simulink model "bh_zaz"  (R2019b)
settings: Solver=ode15s  StartTime=0.0  StopTime=6  FixedStep=0.001  MaxStep=0.1  RelTol=1e-5  AbsTol=1e-5  EnableMultiTasking=on
values from neighbouring files (symbols this model uses):
  L1 = 0.4    [bh_4bar_kin_z_analysis_CLS.m]
  L2 = 1.4    [bh_4bar_kin_z_analysis_CLS.m]
  L3 = 1.2    [bh_4bar_kin_z_analysis_CLS.m]
  N = length(THE_DEG_ANG_VEC)    [bh_4bar_kin_z_analysis_CLS.m]
  X = my_stuff_T.theta_deg_vec    [bh_4bar_kin_z_analysis_CLS.m]
undefined symbols (not defined in the file or in its folder): alpha_0_rad, alpha_dot_0_rad, g, H, I_G1, I_G2, I_G3, m1, m2, m3, phi_0_rad, phi_dot_0_rad, theta_0_rad, theta_dot_0_rad, W, Y, Z
libraries: nesl_utility x20, sm_lib x15, bh_4bar_SL_LIB x6, simulink_extras x5
(part 1 of 2)
settings Model: EnablePacing=on  Creator=bhorton  LastModifiedBy=bhorton
settings DataIOCC: LimitDataPoints=on  ReturnWorkspaceOutputs=off
settings OptimizationCC: LifeSpan=inf
settings DebuggingCC: AllowSymbolicDim=off  PregeneratedLibrarySubsystemCodeDiagnostic=none  SFUnexpectedBacktrackingDiag=warning  SFNoUnconditionalDefaultTransitionDiag=warning  SFExecutionAtInitializationDiag=none  ArithmeticOperatorsInVariantConditions=warning
settings SFSimCC: SimUseLocalCustomCode=off  CustomCodeUndefinedFunction=UseInterfaceOnly
settings RTWCC: RTWUseLocalCustomCode=off
settings CodeAppCC: StateflowObjectComments=on
settings GRTTargetCC: TargetLangStandard=C89/C90 (ANSI)  GeneratePreprocessorConditionals=Disable all
settings ConfigComp: CovMetricSettings=dw  CovHtmlReporting=on  CovSaveCumulativeToWorkspaceVar=on  CovSaveSingleToWorkspaceVar=on  CovExternalEMLEnable=off  CovSFcnEnable=off
settings SimscapeCC: SimscapeNominalValues="[{\"value\":\"10\",\"unit\":\"V\"},{\"value\":\"1\",\"unit\":\"A\"},{\"value\":\"10\",\"unit\":\"N*m\"},{\"value\":\"10\",\"unit\":\"bar\"},{\"value\":\"100\",\"unit\":\"kJ/kg\"},{\"value\":\"1\",\"unit\":\"kW\"},{\"value\":\"300\",\"unit\":\"K\"},{\"value\":\"100\",\"unit\":\"cm^3/s\"},{\"value\":\"1\",\"unit\":\"kN\"},{\"value\":\"1\",\"unit\":\"g/cm^3\"},{\"value\":\"1\",\"unit\":\"l\"},{\"value\":\"1\",\"unit\":\"cm^2\"},{\"value\":\"60\",\"unit\":\"Hz\"}]"  SimscapeLogType=all  SimscapeLogDataHistory=10000
settings ConfigurationSet: Description=SimMechanics 2G
settings ExplorerConfigSet: InternalSimMechanicsExplorerSettings="<ExplorerConfiguration><canonicalview>default</canonicalview><AnimationSetting><BasePlaybackSpeed>1.0</BasePlaybackSpeed><PlaybackSpeedFactor>1.0</PlaybackSpeedFactor></AnimationSetting><TilePanel><TileInfo><Tiles Columns=\"1\" Count=\"1\" Rows=\"1\"><Column Weight=\"1\"/><Row Weight=\"1\"/><Tile Height=\"1\" Width=\"1\" X=\"0\" Y=\"0\"/></Tiles></TileInfo><SceneInfo><SceneViewer><BGColor><R>0.60000002384185791</R><G>0.60000002384185791</G><B>0.60000002384185791</B></BGColor><Camera><DoPerspective>off</DoPerspective><Position><X>0.674057005362880823</X><Y>0.451513124756151407</Y><Z>1.11774542835223722</Z></Position><Center><X>0.674057005362880823</X><Y>0.451513124756151407</Y><Z>-0.00200006458294343936</Z></Center><Up><X>0</X><Y>1</Y><Z>-0</Z></Up><ViewLimDist>1</ViewLimDist><YLim>0.872355052534568132</YLim><XLim>1.30853257880185225</XLim></Camera></SceneViewer></SceneInfo></TilePanel><MechEditorPanel><Cameras/><GfxPanelCameraMap/><VideoCreator><PlaybackSpeedRatio>1.0</PlaybackSpeedRatio><FrameRate>30</FrameRate><VideoFormat>Motion JPEG AVI</VideoFormat><FrameSize>auto</FrameSize></VideoCreator></MechEditorPanel></ExplorerConfiguration>"

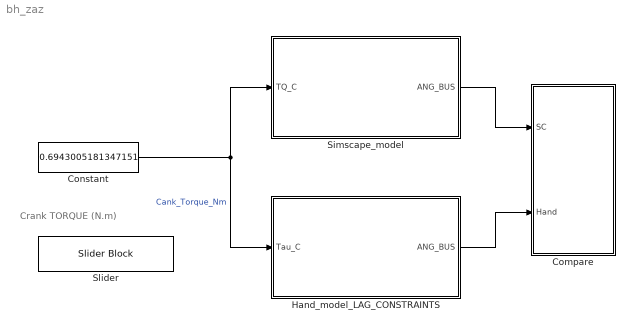
== system bh_zaz ==
  note: Crank TORQUE (N.m)
  Compare : Subsystem
  Constant : Constant  Value=0.6943005181347151
  Hand_model_LAG_CONSTRAINTS : Subsystem
  Simscape_model : Subsystem
  Slider : SliderBlock  ScaleMax=1
  wires:
  Constant/1 -> Simscape_model/1(TQ_C), Hand_model_LAG_CONSTRAINTS/1(Tau_C)  "Cank_Torque_Nm"
  Simscape_model/1(ANG_BUS) -> Compare/1(SC)
  Hand_model_LAG_CONSTRAINTS/1(ANG_BUS) -> Compare/2(Hand)

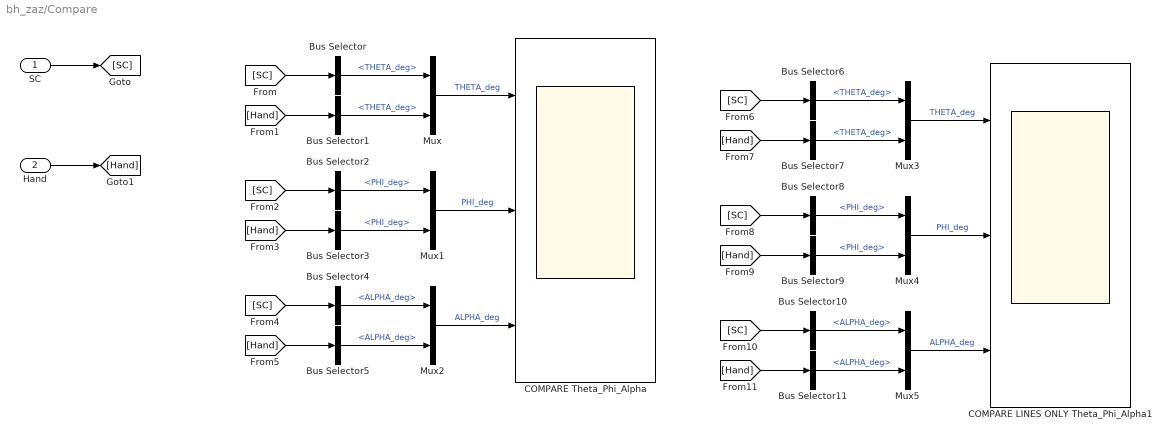
== system bh_zaz/Compare ==
  SC : Inport
  Hand : Inport  Port=2
  Bus Selector{,1,6..7} (4 alike) : BusSelector  OutputSignals=THETA_deg
  Bus Selector{4..5,10..11} (4 alike) : BusSelector  OutputSignals=ALPHA_deg
  Bus Selector{2..3,8..9} (4 alike) : BusSelector  OutputSignals=PHI_deg
  COMPARE LINES ONLY Theta_Phi_Alpha1 : Scope  NumInputPorts=3
  COMPARE Theta_Phi_Alpha : Scope  NumInputPorts=3
  Mux{,1..5} (6 alike) : Mux  Inputs=2
  wires:
  Hand/1 -> [Hand]
  SC/1 -> [SC]
  Mux/1 -> COMPARE Theta_Phi_Alpha/1  "THETA_deg"
  [SC] -> Bus Selector/1
  Bus Selector/1 -> Mux/1  "<THETA_deg>"
  [Hand] -> Bus Selector1/1
  Bus Selector1/1 -> Mux/2  "<THETA_deg>"
  Mux1/1 -> COMPARE Theta_Phi_Alpha/2  "PHI_deg"
  [SC] -> Bus Selector2/1
  Bus Selector3/1 -> Mux1/2  "<PHI_deg>"
  [Hand] -> Bus Selector3/1
  Bus Selector2/1 -> Mux1/1  "<PHI_deg>"
  Mux2/1 -> COMPARE Theta_Phi_Alpha/3  "ALPHA_deg"
  [Hand] -> Bus Selector5/1
  [SC] -> Bus Selector4/1
  Bus Selector5/1 -> Mux2/2  "<ALPHA_deg>"
  Bus Selector4/1 -> Mux2/1  "<ALPHA_deg>"
  Bus Selector10/1 -> Mux5/1  "<ALPHA_deg>"
  [Hand] -> Bus Selector11/1
  Mux5/1 -> COMPARE LINES ONLY Theta_Phi_Alpha1/3  "ALPHA_deg"
  Bus Selector11/1 -> Mux5/2  "<ALPHA_deg>"
  Mux4/1 -> COMPARE LINES ONLY Theta_Phi_Alpha1/2  "PHI_deg"
  [Hand] -> Bus Selector7/1
  Bus Selector8/1 -> Mux4/1  "<PHI_deg>"
  [SC] -> Bus Selector6/1
  Mux3/1 -> COMPARE LINES ONLY Theta_Phi_Alpha1/1  "THETA_deg"
  Bus Selector6/1 -> Mux3/1  "<THETA_deg>"
  [Hand] -> Bus Selector9/1
  [SC] -> Bus Selector8/1
  Bus Selector7/1 -> Mux3/2  "<THETA_deg>"
  [SC] -> Bus Selector10/1
  Bus Selector9/1 -> Mux4/2  "<PHI_deg>"

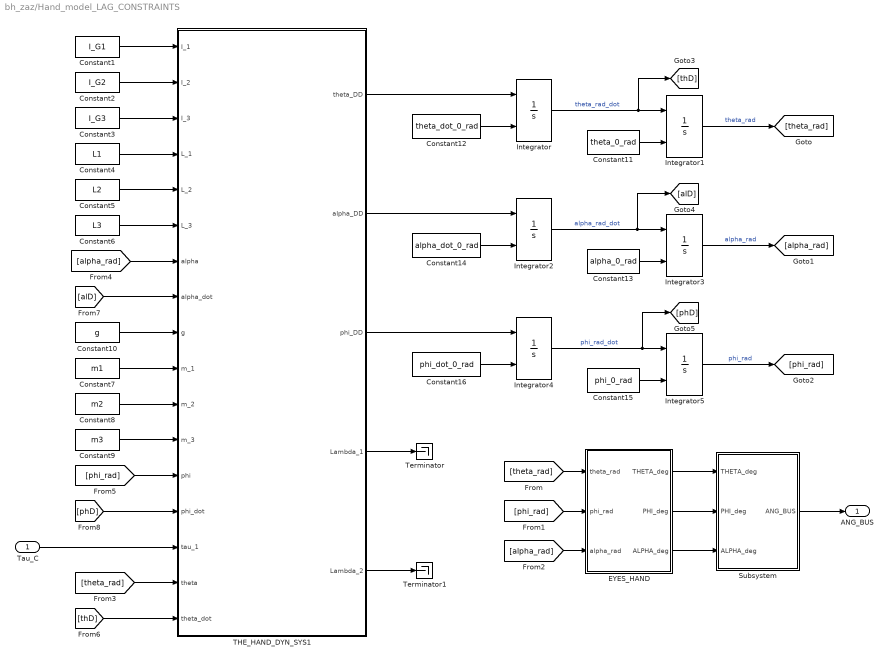
== system bh_zaz/Hand_model_LAG_CONSTRAINTS ==
  Tau_C : Inport
  Constant1 : Constant  Value=I_G1
  Constant10 : Constant  Value=g
  Constant11 : Constant  Value=theta_0_rad
  Constant12 : Constant  Value=theta_dot_0_rad
  Constant13 : Constant  Value=alpha_0_rad
  Constant14 : Constant  Value=alpha_dot_0_rad
  Constant15 : Constant  Value=phi_0_rad
  Constant16 : Constant  Value=phi_dot_0_rad
  Constant2 : Constant  Value=I_G2
  Constant3 : Constant  Value=I_G3
  Constant4 : Constant  Value=L1
  Constant5 : Constant  Value=L2
  Constant6 : Constant  Value=L3
  Constant7 : Constant  Value=m1
  Constant8 : Constant  Value=m2
  Constant9 : Constant  Value=m3
  EYES_HAND : Subsystem
  Integrator{,1..5} (6 alike) : Integrator  InitialConditionSource=external
  Subsystem : Subsystem
  THE_HAND_DYN_SYS1 : MATLAB Function  TreatAsAtomicUnit=on
  Terminator : Terminator
  Terminator1 : Terminator
  ANG_BUS : Outport  VectorParamsAs1DForOutWhenUnconnected=off
  wires:
  Constant7/1 -> THE_HAND_DYN_SYS1/10(m_1)
  Constant8/1 -> THE_HAND_DYN_SYS1/11(m_2)
  Integrator/1 -> [thD], Integrator1/1  "theta_rad_dot"
  Constant6/1 -> THE_HAND_DYN_SYS1/6(L_3)
  Integrator1/1 -> [theta_rad]  "theta_rad"
  Subsystem/1(ANG_BUS) -> ANG_BUS/1
  Constant5/1 -> THE_HAND_DYN_SYS1/5(L_2)
  EYES_HAND/2(PHI_deg) -> Subsystem/2(PHI_deg)
  EYES_HAND/1(THETA_deg) -> Subsystem/1(THETA_deg)
  EYES_HAND/3(ALPHA_deg) -> Subsystem/3(ALPHA_deg)
  [theta_rad] -> EYES_HAND/1(theta_rad)
  [phi_rad] -> EYES_HAND/2(phi_rad)
  THE_HAND_DYN_SYS1/1(theta_DD) -> Integrator/1
  [alpha_rad] -> EYES_HAND/3(alpha_rad)
  Constant3/1 -> THE_HAND_DYN_SYS1/3(I_3)
  Constant2/1 -> THE_HAND_DYN_SYS1/2(I_2)
  Constant4/1 -> THE_HAND_DYN_SYS1/4(L_1)
  Constant10/1 -> THE_HAND_DYN_SYS1/9(g)
  Constant9/1 -> THE_HAND_DYN_SYS1/12(m_3)
  Constant1/1 -> THE_HAND_DYN_SYS1/1(I_1)
  Tau_C/1 -> THE_HAND_DYN_SYS1/15(tau_1)
  Constant12/1 -> Integrator/2
  Constant11/1 -> Integrator1/2
  Integrator2/1 -> [alD], Integrator3/1  "alpha_rad_dot"
  THE_HAND_DYN_SYS1/2(alpha_DD) -> Integrator2/1
  Constant13/1 -> Integrator3/2
  Integrator3/1 -> [alpha_rad]  "alpha_rad"
  Constant14/1 -> Integrator2/2
  Constant15/1 -> Integrator5/2
  Integrator4/1 -> [phD], Integrator5/1  "phi_rad_dot"
  Integrator5/1 -> [phi_rad]  "phi_rad"
  Constant16/1 -> Integrator4/2
  THE_HAND_DYN_SYS1/3(phi_DD) -> Integrator4/1
  THE_HAND_DYN_SYS1/4(Lambda_1) -> Terminator/1
  THE_HAND_DYN_SYS1/5(Lambda_2) -> Terminator1/1
  [theta_rad] -> THE_HAND_DYN_SYS1/16(theta)
  [thD] -> THE_HAND_DYN_SYS1/17(theta_dot)
  [phD] -> THE_HAND_DYN_SYS1/14(phi_dot)
  [phi_rad] -> THE_HAND_DYN_SYS1/13(phi)
  [alD] -> THE_HAND_DYN_SYS1/8(alpha_dot)
  [alpha_rad] -> THE_HAND_DYN_SYS1/7(alpha)

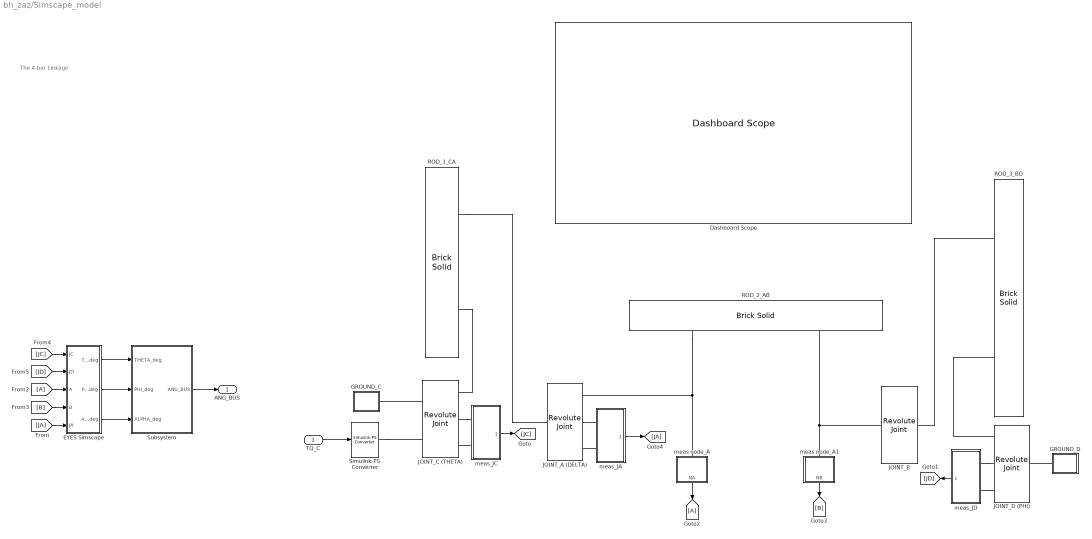
== system bh_zaz/Simscape_model ==
  note: The 4-bar Linkage
  TQ_C : Inport
  Dashboard Scope : DashboardScope
  EYES Simscape : Subsystem
  GROUND_C : Subsystem
  GROUND_D : Subsystem
  JOINT_A (DELTA) : sm_lib/Joints/Revolute Joint  JointMode=Normal  SenseConstraintForce=off  SenseConstraintForceX=off  SenseConstraintForceY=off  SenseConstraintForceZ=off  SenseConstraintTorque=off  SenseConstraintTorqueX=off  SenseConstraintTorqueY=off  SenseConstraintTorqueZ=off  SenseTotalForce=off  SenseTotalForceX=off  SenseTotalForceY=off  SenseTotalForceZ=off  SenseTotalTorque=off  SenseTotalTorqueX=off  SenseTotalTorqueY=off  SenseTotalTorqueZ=off  CompositeWrenchDir=FollowerOnBase  CompositeWrenchFrame=BaseFrame  EquilibriumPosition=0  EquilibriumPositionUnits=deg  SpringStiffness=0  SpringStiffnessUnits=N*m/deg  DampingCoefficient=0  DampingCoefficientUnits=N*m/(deg/s)  TorqueActuationMode=NoTorque  MotionActuationMode=ComputedMotion  SensePosition=on  SenseVelocity=on  SenseAcceleration=off  SenseTorqueForce=off  SenseLowerLimitTorqueForce=off  SenseUpperLimitTorqueForce=off  LowerLimitSpecify=off  LowerLimitBound=-90  LowerLimitBoundUnits=deg  LowerLimitStiffness=1e4  LowerLimitStiffnessUnits=N*m/deg  LowerLimitDamping=10  LowerLimitDampingUnits=N*m/(deg/s)  LowerLimitTransitionRegionWidth=0.1  LowerLimitTransitionRegionWidthUnits=deg  UpperLimitSpecify=off  UpperLimitBound=90  UpperLimitBoundUnits=deg  UpperLimitStiffness=1e4  UpperLimitStiffnessUnits=N*m/deg  UpperLimitDamping=10  UpperLimitDampingUnits=N*m/(deg/s)  UpperLimitTransitionRegionWidth=0.1  UpperLimitTransitionRegionWidthUnits=deg  PositionTargetSpecify=off  PositionTargetPriority=High  PositionTargetValue=0  PositionTargetValueUnits=deg  VelocityTargetSpecify=off  VelocityTargetPriority=High  VelocityTargetValue=0  VelocityTargetValueUnits=deg/s
  JOINT_B : sm_lib/Joints/Revolute Joint  JointMode=Normal  SenseConstraintForce=off  SenseConstraintForceX=off  SenseConstraintForceY=off  SenseConstraintForceZ=off  SenseConstraintTorque=off  SenseConstraintTorqueX=off  SenseConstraintTorqueY=off  SenseConstraintTorqueZ=off  SenseTotalForce=off  SenseTotalForceX=off  SenseTotalForceY=off  SenseTotalForceZ=off  SenseTotalTorque=off  SenseTotalTorqueX=off  SenseTotalTorqueY=off  SenseTotalTorqueZ=off  CompositeWrenchDir=FollowerOnBase  CompositeWrenchFrame=BaseFrame  EquilibriumPosition=0  EquilibriumPositionUnits=deg  SpringStiffness=0  SpringStiffnessUnits=N*m/deg  DampingCoefficient=0  DampingCoefficientUnits=N*m/(deg/s)  TorqueActuationMode=NoTorque  MotionActuationMode=ComputedMotion  SensePosition=off  SenseVelocity=off  SenseAcceleration=off  SenseTorqueForce=off  SenseLowerLimitTorqueForce=off  SenseUpperLimitTorqueForce=off  LowerLimitSpecify=off  LowerLimitBound=-90  LowerLimitBoundUnits=deg  LowerLimitStiffness=1e4  LowerLimitStiffnessUnits=N*m/deg  LowerLimitDamping=10  LowerLimitDampingUnits=N*m/(deg/s)  LowerLimitTransitionRegionWidth=0.1  LowerLimitTransitionRegionWidthUnits=deg  UpperLimitSpecify=off  UpperLimitBound=90  UpperLimitBoundUnits=deg  UpperLimitStiffness=1e4  UpperLimitStiffnessUnits=N*m/deg  UpperLimitDamping=10  UpperLimitDampingUnits=N*m/(deg/s)  UpperLimitTransitionRegionWidth=0.1  UpperLimitTransitionRegionWidthUnits=deg  PositionTargetSpecify=off  PositionTargetPriority=High  PositionTargetValue=0  PositionTargetValueUnits=deg  VelocityTargetSpecify=off  VelocityTargetPriority=High  VelocityTargetValue=0  VelocityTargetValueUnits=deg/s
  JOINT_C (THETA) : sm_lib/Joints/Revolute Joint  JointMode=Normal  SenseConstraintForce=off  SenseConstraintForceX=off  SenseConstraintForceY=off  SenseConstraintForceZ=off  SenseConstraintTorque=off  SenseConstraintTorqueX=off  SenseConstraintTorqueY=off  SenseConstraintTorqueZ=off  SenseTotalForce=off  SenseTotalForceX=off  SenseTotalForceY=off  SenseTotalForceZ=off  SenseTotalTorque=off  SenseTotalTorqueX=off  SenseTotalTorqueY=off  SenseTotalTorqueZ=off  CompositeWrenchDir=FollowerOnBase  CompositeWrenchFrame=BaseFrame  EquilibriumPosition=0  EquilibriumPositionUnits=deg  SpringStiffness=0  SpringStiffnessUnits=N*m/deg  DampingCoefficient=0  DampingCoefficientUnits=N*m/(deg/s)  TorqueActuationMode=InputTorque  MotionActuationMode=ComputedMotion  SensePosition=on  SenseVelocity=on  SenseAcceleration=off  SenseTorqueForce=off  SenseLowerLimitTorqueForce=off  SenseUpperLimitTorqueForce=off  LowerLimitSpecify=off  LowerLimitBound=-90  LowerLimitBoundUnits=deg  LowerLimitStiffness=1e4  LowerLimitStiffnessUnits=N*m/deg  LowerLimitDamping=10  LowerLimitDampingUnits=N*m/(deg/s)  LowerLimitTransitionRegionWidth=0.1  LowerLimitTransitionRegionWidthUnits=deg  UpperLimitSpecify=off  UpperLimitBound=90  UpperLimitBoundUnits=deg  UpperLimitStiffness=1e4  UpperLimitStiffnessUnits=N*m/deg  UpperLimitDamping=10  UpperLimitDampingUnits=N*m/(deg/s)  UpperLimitTransitionRegionWidth=0.1  UpperLimitTransitionRegionWidthUnits=deg  PositionTargetSpecify=on  PositionTargetPriority=High  PositionTargetValue=joints.C.ang_degs  PositionTargetValueUnits=deg  VelocityTargetSpecify=on  VelocityTargetPriority=High  VelocityTargetValue=joints.C.vel_degs  VelocityTargetValueUnits=deg/s
      settings: AttributesFormatString=|
      | init_pos =%<PositionTargetValue>
      | %<PositionTargetValueUnits>
      | init_VEL =
      | %<VelocityTargetValue>
      | %<VelocityTargetValueUnits>
  JOINT_D (PHI) : sm_lib/Joints/Revolute Joint  JointMode=Normal  SenseConstraintForce=off  SenseConstraintForceX=off  SenseConstraintForceY=off  SenseConstraintForceZ=off  SenseConstraintTorque=off  SenseConstraintTorqueX=off  SenseConstraintTorqueY=off  SenseConstraintTorqueZ=off  SenseTotalForce=off  SenseTotalForceX=off  SenseTotalForceY=off  SenseTotalForceZ=off  SenseTotalTorque=off  SenseTotalTorqueX=off  SenseTotalTorqueY=off  SenseTotalTorqueZ=off  CompositeWrenchDir=FollowerOnBase  CompositeWrenchFrame=BaseFrame  EquilibriumPosition=0  EquilibriumPositionUnits=deg  SpringStiffness=0  SpringStiffnessUnits=N*m/deg  DampingCoefficient=0  DampingCoefficientUnits=N*m/(deg/s)  TorqueActuationMode=NoTorque  MotionActuationMode=ComputedMotion  SensePosition=on  SenseVelocity=on  SenseAcceleration=off  SenseTorqueForce=off  SenseLowerLimitTorqueForce=off  SenseUpperLimitTorqueForce=off  LowerLimitSpecify=off  LowerLimitBound=-90  LowerLimitBoundUnits=deg  LowerLimitStiffness=1e4  LowerLimitStiffnessUnits=N*m/deg  LowerLimitDamping=10  LowerLimitDampingUnits=N*m/(deg/s)  LowerLimitTransitionRegionWidth=0.1  LowerLimitTransitionRegionWidthUnits=deg  UpperLimitSpecify=off  UpperLimitBound=90  UpperLimitBoundUnits=deg  UpperLimitStiffness=1e4  UpperLimitStiffnessUnits=N*m/deg  UpperLimitDamping=10  UpperLimitDampingUnits=N*m/(deg/s)  UpperLimitTransitionRegionWidth=0.1  UpperLimitTransitionRegionWidthUnits=deg  PositionTargetSpecify=on  PositionTargetPriority=High  PositionTargetValue=joints.D.ang_degs  PositionTargetValueUnits=deg  VelocityTargetSpecify=off  VelocityTargetPriority=High  VelocityTargetValue=0  VelocityTargetValueUnits=deg/s
      settings: AttributesFormatString=|
      | init_pos =%<PositionTargetValue>
      | %<PositionTargetValueUnits>
  ROD_1_CA : sm_lib/Body Elements/Brick Solid  GraphicAmbientColor=[0.15 0.15 0.15 1.0]  BasedOnType=Density  BrickDimensions=[L1,H,W]  BrickDimensionUnits=m  CenterOfMass=[0 0 0]  CenterOfMassUnits=m  GraphicDiffuseColor=[1.0 0.4 0.6]  Density=density  DensityUnits=kg/m^3  DoExposeReferenceFrame=on  GraphicEmissiveColor=[0.0 0.0 0.0 1.0]  ExportEntireGeometry=off  SerializedFrames=<Frames><Frame><Id>Frame2</Id><Value><Name>A</Name><Origin><Source>GeometricFeature</Source><FeatureName>+z +x curve</FeatureName></Origin><PrimaryAxis><DefinedDirection>+Z</DefinedDirection><Source>ReferenceFrame</Source><SourceDirection>+Z</SourceDirection><FeatureName></FeatureName></PrimaryAxis><SecondaryAxis><DefinedDirection>+X</DefinedDirection><Source>ReferenceFrame</Source><SourceDirection>+X</SourceDirection><FeatureName></FeatureName></SecondaryAxis></Value></Frame><Frame><Id>Frame3</Id><Value><Name>C</Name><Origin><Source>GeometricFeature</Source><FeatureName>+z -x curve</FeatureName></Origin><PrimaryAxis><DefinedDirection>+Z</DefinedDirection><Source>ReferenceFrame</Source><SourceDirection>+Z</SourceDirection><FeatureName></FeatureName></PrimaryAxis><SecondaryAxis><DefinedDirection>+X</DefinedDirection><Source>ReferenceFrame</Source><SourceDirection>+X</SourceDirection><FeatureName></FeatureName></SecondaryAxis></Value></Frame></Frames>  MarkerShape=Sphere  MarkerSize=10  GraphicType=FromGeometry  InertiaType=CalculateFromGeometry  Mass=1  MassUnits=kg  MomentsOfInertia=[1 1 1]  MomentsOfInertiaUnits=kg*m^2  GraphicOpacity=1.0  ProductsOfInertia=[0 0 0]  ProductsOfInertiaUnits=kg*m^2  GraphicShininess=75  GraphicSpecularColor=[0.5 0.5 0.5 1.0]  GraphicVisPropType=SimpleVisualProperties
  ROD_2_AB : sm_lib/Body Elements/Brick Solid  GraphicAmbientColor=[0.15 0.15 0.15 1.0]  BasedOnType=Density  BrickDimensions=[L2,H,W]  BrickDimensionUnits=m  CenterOfMass=[0 0 0]  CenterOfMassUnits=m  GraphicDiffuseColor=[0.0 1.0 0.2]  Density=density  DensityUnits=kg/m^3  DoExposeReferenceFrame=on  GraphicEmissiveColor=[0.0 0.0 0.0 1.0]  ExportEntireGeometry=off  SerializedFrames=<Frames><Frame><Id>Frame1</Id><Value><Name>A</Name><Origin><Source>GeometricFeature</Source><FeatureName>+z -x curve</FeatureName></Origin><PrimaryAxis><DefinedDirection>+Z</DefinedDirection><Source>ReferenceFrame</Source><SourceDirection>+Z</SourceDirection><FeatureName></FeatureName></PrimaryAxis><SecondaryAxis><DefinedDirection>+X</DefinedDirection><Source>ReferenceFrame</Source><SourceDirection>+X</SourceDirection><FeatureName></FeatureName></SecondaryAxis></Value></Frame><Frame><Id>Frame2</Id><Value><Name>B</Name><Origin><Source>GeometricFeature</Source><FeatureName>+z +x curve</FeatureName></Origin><PrimaryAxis><DefinedDirection>+Z</DefinedDirection><Source>ReferenceFrame</Source><SourceDirection>+Z</SourceDirection><FeatureName></FeatureName></PrimaryAxis><SecondaryAxis><DefinedDirection>+X</DefinedDirection><Source>ReferenceFrame</Source><SourceDirection>+X</SourceDirection><FeatureName></FeatureName></SecondaryAxis></Value></Frame></Frames>  MarkerShape=Sphere  MarkerSize=10  GraphicType=FromGeometry  InertiaType=CalculateFromGeometry  Mass=1  MassUnits=kg  MomentsOfInertia=[1 1 1]  MomentsOfInertiaUnits=kg*m^2  GraphicOpacity=1.0  ProductsOfInertia=[0 0 0]  ProductsOfInertiaUnits=kg*m^2  GraphicShininess=75  GraphicSpecularColor=[0.5 0.5 0.5 1.0]  GraphicVisPropType=SimpleVisualProperties
  ROD_3_BD : sm_lib/Body Elements/Brick Solid  GraphicAmbientColor=[0.15 0.15 0.15 1.0]  BasedOnType=Density  BrickDimensions=[L3,H,W]  BrickDimensionUnits=m  CenterOfMass=[0 0 0]  CenterOfMassUnits=m  GraphicDiffuseColor=[0.2 0.2 1.0]  Density=density  DensityUnits=kg/m^3  DoExposeReferenceFrame=on  GraphicEmissiveColor=[0.0 0.0 0.0 1.0]  ExportEntireGeometry=off  SerializedFrames=<Frames><Frame><Id>Frame1</Id><Value><Name>B</Name><Origin><Source>GeometricFeature</Source><FeatureName>+z +x curve</FeatureName></Origin><PrimaryAxis><DefinedDirection>+Z</DefinedDirection><Source>ReferenceFrame</Source><SourceDirection>+Z</SourceDirection><FeatureName></FeatureName></PrimaryAxis><SecondaryAxis><DefinedDirection>+X</DefinedDirection><Source>ReferenceFrame</Source><SourceDirection>+X</SourceDirection><FeatureName></FeatureName></SecondaryAxis></Value></Frame><Frame><Id>Frame2</Id><Value><Name>D</Name><Origin><Source>GeometricFeature</Source><FeatureName>+z -x curve</FeatureName></Origin><PrimaryAxis><DefinedDirection>+Z</DefinedDirection><Source>ReferenceFrame</Source><SourceDirection>+Z</SourceDirection><FeatureName></FeatureName></PrimaryAxis><SecondaryAxis><DefinedDirection>+X</DefinedDirection><Source>ReferenceFrame</Source><SourceDirection>+X</SourceDirection><FeatureName></FeatureName></SecondaryAxis></Value></Frame></Frames>  MarkerShape=Sphere  MarkerSize=10  GraphicType=FromGeometry  InertiaType=CalculateFromGeometry  Mass=1  MassUnits=kg  MomentsOfInertia=[1 1 1]  MomentsOfInertiaUnits=kg*m^2  GraphicOpacity=1.0  ProductsOfInertia=[0 0 0]  ProductsOfInertiaUnits=kg*m^2  GraphicShininess=75  GraphicSpecularColor=[0.5 0.5 0.5 1.0]  GraphicVisPropType=SimpleVisualProperties
  Simulink-PS Converter : nesl_utility/Simulink-PS Converter  PhysicalDomain=network_engine_domain  SubClassName=ps_input  LeftPortType=input  RightPortType=output  PseudoPeriodic=off  Frequencies=[]  NoiseDistribution=none  NoiseParameters=[]  Unit=N*m  AffineConversion=off  FilteringAndDerivatives=filter  SimscapeFilterOrder=1  InputFilterTimeConstant=0.001  UdotUserProvided=2
  Subsystem : Subsystem
  meas node_A : Subsystem
  meas node_A1 : Subsystem
  meas_JA : Subsystem
  meas_JC : Subsystem
  meas_JD : Subsystem
  ANG_BUS : Outport  VectorParamsAs1DForOutWhenUnconnected=off
  wires:
  [JC] -> EYES Simscape/1(JC)
  meas_JC/1(PV_BUS) -> [JC]
  [JA] -> EYES Simscape/5(JA)
  [B] -> EYES Simscape/4(B)
  EYES Simscape/3(ALPHA_deg) -> Subsystem/3(ALPHA_deg)
  TQ_C/1 -> Simulink-PS Converter/1
  [JD] -> EYES Simscape/2(JD)
  [A] -> EYES Simscape/3(A)
  meas_JA/1(PV_BUS) -> [JA]
  EYES Simscape/1(THETA_deg) -> Subsystem/1(THETA_deg)
  meas_JD/1(PV_BUS) -> [JD]
  EYES Simscape/2(PHI_deg) -> Subsystem/2(PHI_deg)
  Subsystem/1(ANG_BUS) -> ANG_BUS/1
  meas node_A/1(NA) -> [A]
  meas node_A1/1(NB) -> [B]
  connections:
  meas_JD/LConn2 -- JOINT_D (PHI)/RConn3
  JOINT_D (PHI)/RConn1 -- ROD_3_BD/LConn2
  JOINT_C (THETA)/LConn1 -- GROUND_C/RConn1
  meas_JA/LConn1 -- JOINT_A (DELTA)/RConn2
  meas_JD/LConn1 -- JOINT_D (PHI)/RConn2
  ROD_3_BD/LConn1 -- JOINT_B/RConn1
  meas_JA/LConn2 -- JOINT_A (DELTA)/RConn3
  GROUND_D/RConn1 -- JOINT_D (PHI)/LConn1
  JOINT_C (THETA)/RConn2 -- meas_JC/LConn1
  ROD_2_AB/LConn1 -- meas node_A/LConn1 -- JOINT_A (DELTA)/RConn1
  ROD_1_CA/LConn2 -- JOINT_C (THETA)/RConn1
  Simulink-PS Converter/RConn1 -- JOINT_C (THETA)/LConn2
  meas_JC/LConn2 -- JOINT_C (THETA)/RConn3
  ROD_1_CA/LConn1 -- JOINT_A (DELTA)/LConn1
  JOINT_B/LConn1 -- meas node_A1/LConn1 -- ROD_2_AB/LConn2

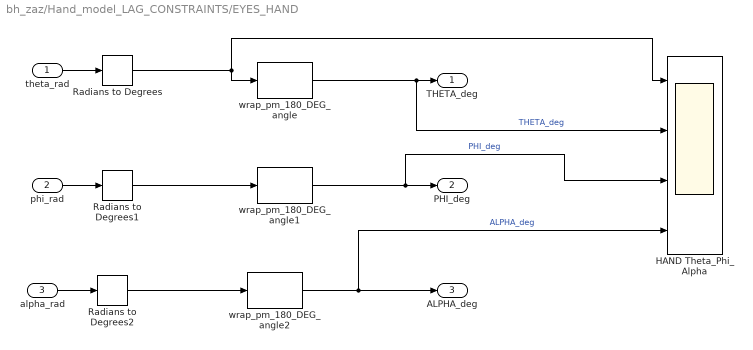
== system bh_zaz/Hand_model_LAG_CONSTRAINTS/EYES_HAND ==
  theta_rad : Inport
  phi_rad : Inport  Port=2
  alpha_rad : Inport  Port=3
  HAND Theta_Phi_Alpha : Scope  NumInputPorts=4
  Radians to Degrees : simulink_extras/Transformations/Radians to Degrees
  Radians to Degrees1 : simulink_extras/Transformations/Radians to Degrees
  Radians to Degrees2 : simulink_extras/Transformations/Radians to Degrees
  wrap_pm_180_DEG_angle : bh_4bar_SL_LIB/4bar_basics/wrap_pm_180_DEG_angle  SystemSampleTime=-1  Latency=0  AutoFrameSizeCalculation=off
  wrap_pm_180_DEG_angle1 : bh_4bar_SL_LIB/4bar_basics/wrap_pm_180_DEG_angle  SystemSampleTime=-1  Latency=0  AutoFrameSizeCalculation=off
  wrap_pm_180_DEG_angle2 : bh_4bar_SL_LIB/4bar_basics/wrap_pm_180_DEG_angle  SystemSampleTime=-1  Latency=0  AutoFrameSizeCalculation=off
  THETA_deg : Outport  VectorParamsAs1DForOutWhenUnconnected=off
  PHI_deg : Outport  Port=2  VectorParamsAs1DForOutWhenUnconnected=off
  ALPHA_deg : Outport  Port=3  VectorParamsAs1DForOutWhenUnconnected=off
  wires:
  theta_rad/1 -> Radians to Degrees/1
  alpha_rad/1 -> Radians to Degrees2/1
  phi_rad/1 -> Radians to Degrees1/1
  Radians to Degrees/1 -> wrap_pm_180_DEG_angle/1, HAND Theta_Phi_Alpha/1
  Radians to Degrees1/1 -> wrap_pm_180_DEG_angle1/1
  Radians to Degrees2/1 -> wrap_pm_180_DEG_angle2/1
  wrap_pm_180_DEG_angle/1 -> HAND Theta_Phi_Alpha/2, THETA_deg/1  "THETA_deg"
  wrap_pm_180_DEG_angle1/1 -> HAND Theta_Phi_Alpha/3, PHI_deg/1  "PHI_deg"
  wrap_pm_180_DEG_angle2/1 -> HAND Theta_Phi_Alpha/4, ALPHA_deg/1  "ALPHA_deg"

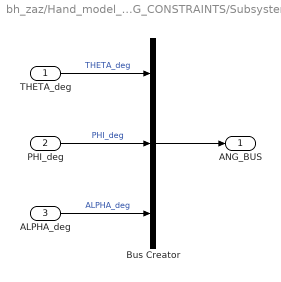
== system bh_zaz/Hand_model_LAG_CONSTRAINTS/Subsystem ==
  THETA_deg : Inport
  PHI_deg : Inport  Port=2
  ALPHA_deg : Inport  Port=3
  Bus Creator : BusCreator  Inputs=3
  ANG_BUS : Outport  VectorParamsAs1DForOutWhenUnconnected=off
  wires:
  ALPHA_deg/1 -> Bus Creator/3  "ALPHA_deg"
  PHI_deg/1 -> Bus Creator/2  "PHI_deg"
  THETA_deg/1 -> Bus Creator/1  "THETA_deg"
  Bus Creator/1 -> ANG_BUS/1

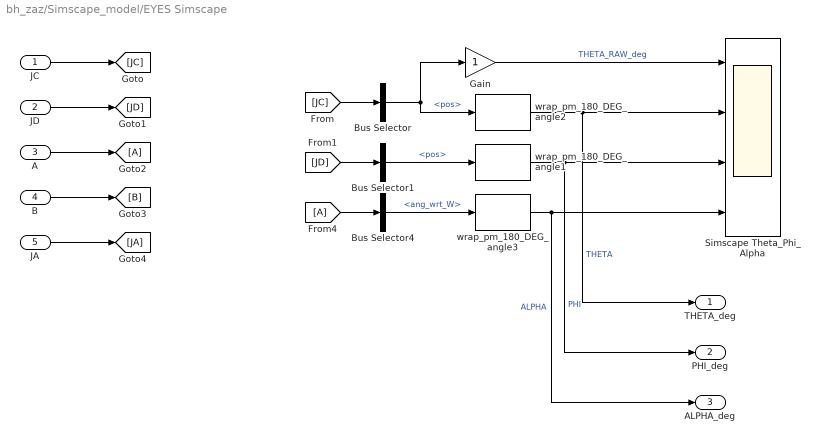
== system bh_zaz/Simscape_model/EYES Simscape ==
  JC : Inport
  JD : Inport  Port=2
  A : Inport  Port=3
  B : Inport  Port=4
  JA : Inport  Port=5
  Bus Selector : BusSelector  OutputSignals=pos
  Bus Selector1 : BusSelector  OutputSignals=pos
  Bus Selector4 : BusSelector  OutputSignals=ang_wrt_W
  Gain : Gain
  Simscape Theta_Phi_Alpha : Scope  NumInputPorts=4
  wrap_pm_180_DEG_angle1 : bh_4bar_SL_LIB/4bar_basics/wrap_pm_180_DEG_angle  SystemSampleTime=-1  Latency=0  AutoFrameSizeCalculation=off
  wrap_pm_180_DEG_angle2 : bh_4bar_SL_LIB/4bar_basics/wrap_pm_180_DEG_angle  SystemSampleTime=-1  Latency=0  AutoFrameSizeCalculation=off
  wrap_pm_180_DEG_angle3 : bh_4bar_SL_LIB/4bar_basics/wrap_pm_180_DEG_angle  SystemSampleTime=-1  Latency=0  AutoFrameSizeCalculation=off
  THETA_deg : Outport  VectorParamsAs1DForOutWhenUnconnected=off
  PHI_deg : Outport  Port=2  VectorParamsAs1DForOutWhenUnconnected=off
  ALPHA_deg : Outport  Port=3  VectorParamsAs1DForOutWhenUnconnected=off
  wires:
  B/1 -> [B]
  A/1 -> [A]
  JD/1 -> [JD]
  JC/1 -> [JC]
  [JD] -> Bus Selector1/1
  [JC] -> Bus Selector/1
  Bus Selector/1 -> wrap_pm_180_DEG_angle2/1, Gain/1  "<pos>"
  [A] -> Bus Selector4/1
  wrap_pm_180_DEG_angle2/1 -> THETA_deg/1, Simscape Theta_Phi_Alpha/2  "THETA"
  wrap_pm_180_DEG_angle1/1 -> PHI_deg/1, Simscape Theta_Phi_Alpha/3  "PHI"
  JA/1 -> [JA]
  wrap_pm_180_DEG_angle3/1 -> ALPHA_deg/1, Simscape Theta_Phi_Alpha/4  "ALPHA"
  Gain/1 -> Simscape Theta_Phi_Alpha/1  "THETA_RAW_deg"
  Bus Selector1/1 -> wrap_pm_180_DEG_angle1/1  "<pos>"
  Bus Selector4/1 -> wrap_pm_180_DEG_angle3/1  "<ang_wrt_W>"

== system bh_zaz/Simscape_model/GROUND_C ==
  Mechanism Configuration : sm_lib/Utilities/Mechanism Configuration  UniformGravity=Constant  GravityVector="[0 -g  0]"  GravityUnits=m/s^2  LinearizationDelta=0.001
  Solver Configuration : nesl_utility/Solver Configuration  PhysicalDomain=network_engine_domain  SubClassName=solver  LeftPortType=input  RightPortType=generic  Tones=[]  Harmonics=[]  SimulateNoise=off  Profile=off  UseLocalSampling=off  EnableSwitchedLinearOptims=on  FrequencyDomain=off  UseCCode=off  RelTol=0.001  AbsTol=1e-06  MinStep=1e-09  ToWorkspace=off  RevertToSquareIcSolve=off  NumHomotopyIterations=100  PhasorMode=off  PhasorModeNumHarmonics=1  DoDC=off  ResidualTolerance=1e-09  UseLocalSolver=off  LocalSolverChoice=NE_BACKWARD_EULER_ADVANCER  LocalSolverSampleTime=0.001  DoFixedCost=off  MaxNonlinIter=3  MaxModeIter=2  LinearAlgebra=Sparse  EquationFormulation=NE_TIME_EF  DelaysMemoryBudget=1024  AutomaticFiltering=on  FilteringTimeConstant=0.001  PartitionStorageMethod=AS_NEEDED  PartitionMemoryBudget=1024  PartitionMethod=FAST
  World Frame : sm_lib/Frames and Transforms/World Frame
  Conn1 : PMIOPort  Side=Right
  connections:
  Solver Configuration/RConn1 -- Conn1/RConn1 -- Mechanism Configuration/RConn1 -- World Frame/RConn1

== system bh_zaz/Simscape_model/GROUND_D ==
  Rigid Transform : sm_lib/Frames and Transforms/Rigid Transform  TranslationMethod=StandardAxis  TranslationStandardOffset=L4  TranslationLengthUnit=m  TranslationStandardAxis=+X  TranslationCartesianOffset=[0 0 0]  TranslationROffset=0  TranslationROffsetUnits=m  TranslationZOffset=0  TranslationZOffsetUnits=m  TranslationThetaOffset=0  TranslationThetaOffsetUnits=deg  RotationMethod=None  RotationAngleUnits=deg  RotationStandardAxis=+Z  RotationAngle=0.0  RotationArbitraryAxis=[0 0 1]  FollAlignAxisA=+X  BaseAlignAxisA=+Y  FollAlignAxisB=+Y  BaseAlignAxisB=+Z  RotationSequenceAxes=FollowerAxes  RotationSequence=XYX  RotationSequenceAngles=[0 0 0]  RotationSequenceAnglesUnits=deg  RotationMatrix=[1 0 0; 0 1 0; 0 0 1]
  World Frame1 : sm_lib/Frames and Transforms/World Frame
  Conn1 : PMIOPort  Side=Right
  connections:
  Rigid Transform/LConn1 -- World Frame1/RConn1
  Rigid Transform/RConn1 -- Conn1/RConn1

== system bh_zaz/Simscape_model/Subsystem ==
  THETA_deg : Inport
  PHI_deg : Inport  Port=2
  ALPHA_deg : Inport  Port=3
  Bus Creator : BusCreator  Inputs=3
  ANG_BUS : Outport  VectorParamsAs1DForOutWhenUnconnected=off
  wires:
  ALPHA_deg/1 -> Bus Creator/3  "ALPHA_deg"
  PHI_deg/1 -> Bus Creator/2  "PHI_deg"
  THETA_deg/1 -> Bus Creator/1  "THETA_deg"
  Bus Creator/1 -> ANG_BUS/1

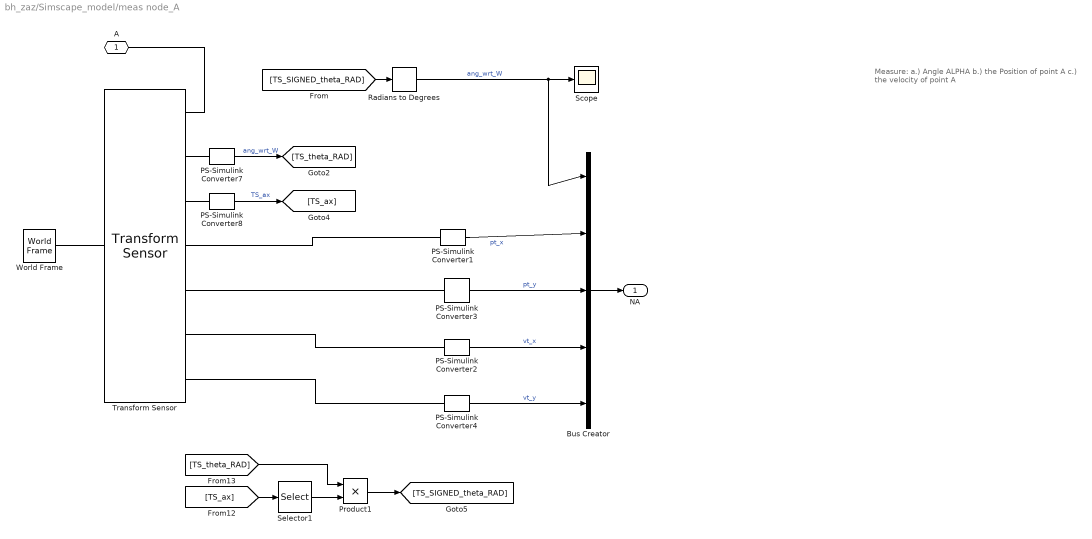
== system bh_zaz/Simscape_model/meas node_A ==
  note: Measure:
      | a.) Angle ALPHA
      | b.) the Position of point A
      | c.) the velocity of point A
  Bus Creator : BusCreator  Inputs=5
  PS-Simulink Converter1 : nesl_utility/PS-Simulink Converter  PhysicalDomain=network_engine_domain  SubClassName=ps_output  LeftPortType=input  RightPortType=output  PseudoPeriodic=off  Frequencies=[]  Unit=m  AffineConversion=off
      settings: AttributesFormatString=UNITS=%<Unit>
  PS-Simulink Converter2 : nesl_utility/PS-Simulink Converter  PhysicalDomain=network_engine_domain  SubClassName=ps_output  LeftPortType=input  RightPortType=output  PseudoPeriodic=off  Frequencies=[]  Unit=m/s  AffineConversion=off
      settings: AttributesFormatString=UNITS=%<Unit>
  PS-Simulink Converter3 : nesl_utility/PS-Simulink Converter  PhysicalDomain=network_engine_domain  SubClassName=ps_output  LeftPortType=input  RightPortType=output  PseudoPeriodic=off  Frequencies=[]  Unit=m  AffineConversion=off
      settings: AttributesFormatString=UNITS=%<Unit>
  PS-Simulink Converter4 : nesl_utility/PS-Simulink Converter  PhysicalDomain=network_engine_domain  SubClassName=ps_output  LeftPortType=input  RightPortType=output  PseudoPeriodic=off  Frequencies=[]  Unit=m/s  AffineConversion=off
      settings: AttributesFormatString=UNITS=%<Unit>
  PS-Simulink Converter7 : nesl_utility/PS-Simulink Converter  PhysicalDomain=network_engine_domain  SubClassName=ps_output  LeftPortType=input  RightPortType=output  PseudoPeriodic=off  Frequencies=[]  Unit=rad  AffineConversion=off
      settings: AttributesFormatString=UNITS=%<Unit>
  PS-Simulink Converter8 : nesl_utility/PS-Simulink Converter  PhysicalDomain=network_engine_domain  SubClassName=ps_output  LeftPortType=input  RightPortType=output  PseudoPeriodic=off  Frequencies=[]  Unit=1  AffineConversion=off
      settings: AttributesFormatString=UNITS=%<Unit>
  Product1 : Product
  Radians to Degrees : simulink_extras/Transformations/Radians to Degrees
  Scope : Scope
  Selector1 : Selector  InputPortWidth=3  IndexOptions=Index vector (dialog)  Indices=3  OutputSizes=1
  Transform Sensor : sm_lib/Frames and Transforms/Transform Sensor  MeasurementFrame=World  SenseAngle=on  SenseAxis=on  SenseAngle1=off  SenseAngle2=off  SenseAngle3=off  SenseQ=off  SenseR=off  SenseOmegaX=off  SenseOmegaY=off  SenseOmegaZ=off  SenseOmega1=off  SenseOmega2=off  SenseOmega3=off  SenseQDot=off  SenseRDot=off  SenseAlphaX=off  SenseAlphaY=off  SenseAlphaZ=off  SenseAlpha1=off  SenseAlpha2=off  SenseAlpha3=off  SenseQDDot=off  SenseRDDot=off  SenseX=on  SenseY=on  SenseZ=off  SenseRad=off  SenseAzim=off  SenseDist=off  SenseInc=off  SenseXDot=on  SenseYDot=on  SenseZDot=off  SenseRadDot=off  SenseAzimDot=off  SenseDistDot=off  SenseIncDot=off  SenseXDDot=off  SenseYDDot=off  SenseZDDot=off  SenseRadDDot=off  SenseAzimDDot=off  SenseDistDDot=off  SenseIncDDot=off
  World Frame : sm_lib/Frames and Transforms/World Frame
  A : PMIOPort  Side=Left
  NA : Outport  VectorParamsAs1DForOutWhenUnconnected=off
  wires:
  PS-Simulink Converter2/1 -> Bus Creator/4  "vt_x"
  Bus Creator/1 -> NA/1
  PS-Simulink Converter1/1 -> Bus Creator/2  "pt_x"
  PS-Simulink Converter4/1 -> Bus Creator/5  "vt_y"
  PS-Simulink Converter3/1 -> Bus Creator/3  "pt_y"
  Radians to Degrees/1 -> Bus Creator/1, Scope/1  "ang_wrt_W"
  [TS_theta_RAD] -> Product1/1
  [TS_ax] -> Selector1/1
  Product1/1 -> [TS_SIGNED_theta_RAD]
  Selector1/1 -> Product1/2
  PS-Simulink Converter7/1 -> [TS_theta_RAD]  "ang_wrt_W"
  PS-Simulink Converter8/1 -> [TS_ax]  "TS_ax"
  [TS_SIGNED_theta_RAD] -> Radians to Degrees/1
  connections:
  A/RConn1 -- Transform Sensor/RConn1
  Transform Sensor/LConn1 -- World Frame/RConn1
  Transform Sensor/RConn7 -- PS-Simulink Converter4/LConn1
  PS-Simulink Converter2/LConn1 -- Transform Sensor/RConn6
  PS-Simulink Converter3/LConn1 -- Transform Sensor/RConn5
  PS-Simulink Converter1/LConn1 -- Transform Sensor/RConn4
  PS-Simulink Converter7/LConn1 -- Transform Sensor/RConn2
  PS-Simulink Converter8/LConn1 -- Transform Sensor/RConn3

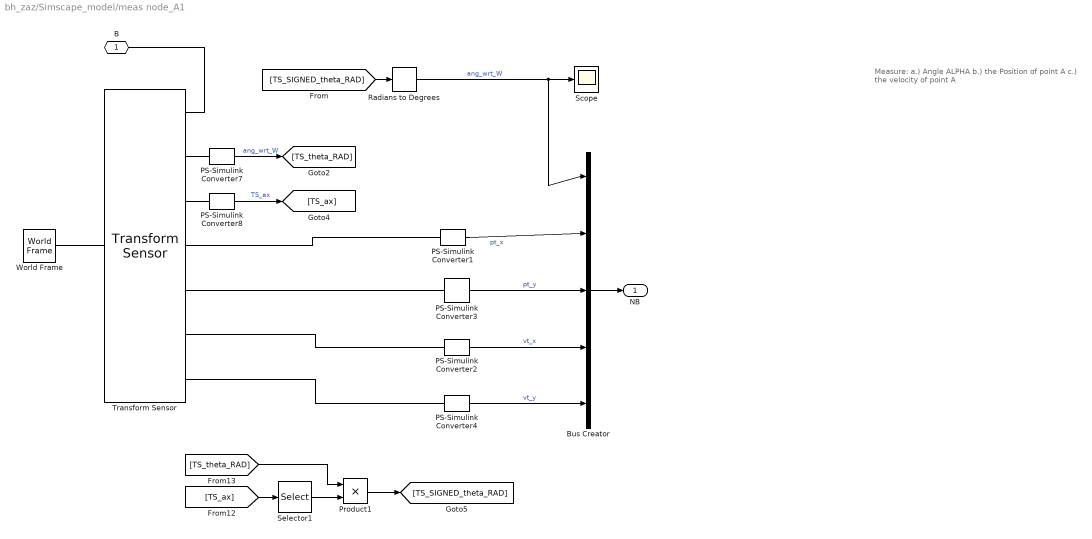
== system bh_zaz/Simscape_model/meas node_A1 ==
  note: Measure:
      | a.) Angle ALPHA
      | b.) the Position of point A
      | c.) the velocity of point A
  Bus Creator : BusCreator  Inputs=5
  PS-Simulink Converter1 : nesl_utility/PS-Simulink Converter  PhysicalDomain=network_engine_domain  SubClassName=ps_output  LeftPortType=input  RightPortType=output  PseudoPeriodic=off  Frequencies=[]  Unit=m  AffineConversion=off
      settings: AttributesFormatString=UNITS=%<Unit>
  PS-Simulink Converter2 : nesl_utility/PS-Simulink Converter  PhysicalDomain=network_engine_domain  SubClassName=ps_output  LeftPortType=input  RightPortType=output  PseudoPeriodic=off  Frequencies=[]  Unit=m/s  AffineConversion=off
      settings: AttributesFormatString=UNITS=%<Unit>
  PS-Simulink Converter3 : nesl_utility/PS-Simulink Converter  PhysicalDomain=network_engine_domain  SubClassName=ps_output  LeftPortType=input  RightPortType=output  PseudoPeriodic=off  Frequencies=[]  Unit=m  AffineConversion=off
      settings: AttributesFormatString=UNITS=%<Unit>
  PS-Simulink Converter4 : nesl_utility/PS-Simulink Converter  PhysicalDomain=network_engine_domain  SubClassName=ps_output  LeftPortType=input  RightPortType=output  PseudoPeriodic=off  Frequencies=[]  Unit=m/s  AffineConversion=off
      settings: AttributesFormatString=UNITS=%<Unit>
  PS-Simulink Converter7 : nesl_utility/PS-Simulink Converter  PhysicalDomain=network_engine_domain  SubClassName=ps_output  LeftPortType=input  RightPortType=output  PseudoPeriodic=off  Frequencies=[]  Unit=rad  AffineConversion=off
      settings: AttributesFormatString=UNITS=%<Unit>
  PS-Simulink Converter8 : nesl_utility/PS-Simulink Converter  PhysicalDomain=network_engine_domain  SubClassName=ps_output  LeftPortType=input  RightPortType=output  PseudoPeriodic=off  Frequencies=[]  Unit=1  AffineConversion=off
      settings: AttributesFormatString=UNITS=%<Unit>
  Product1 : Product
  Radians to Degrees : simulink_extras/Transformations/Radians to Degrees
  Scope : Scope
  Selector1 : Selector  InputPortWidth=3  IndexOptions=Index vector (dialog)  Indices=3  OutputSizes=1
  Transform Sensor : sm_lib/Frames and Transforms/Transform Sensor  MeasurementFrame=World  SenseAngle=on  SenseAxis=on  SenseAngle1=off  SenseAngle2=off  SenseAngle3=off  SenseQ=off  SenseR=off  SenseOmegaX=off  SenseOmegaY=off  SenseOmegaZ=off  SenseOmega1=off  SenseOmega2=off  SenseOmega3=off  SenseQDot=off  SenseRDot=off  SenseAlphaX=off  SenseAlphaY=off  SenseAlphaZ=off  SenseAlpha1=off  SenseAlpha2=off  SenseAlpha3=off  SenseQDDot=off  SenseRDDot=off  SenseX=on  SenseY=on  SenseZ=off  SenseRad=off  SenseAzim=off  SenseDist=off  SenseInc=off  SenseXDot=on  SenseYDot=on  SenseZDot=off  SenseRadDot=off  SenseAzimDot=off  SenseDistDot=off  SenseIncDot=off  SenseXDDot=off  SenseYDDot=off  SenseZDDot=off  SenseRadDDot=off  SenseAzimDDot=off  SenseDistDDot=off  SenseIncDDot=off
  World Frame : sm_lib/Frames and Transforms/World Frame
  B : PMIOPort  Side=Left
  NB : Outport  VectorParamsAs1DForOutWhenUnconnected=off
  wires:
  PS-Simulink Converter2/1 -> Bus Creator/4  "vt_x"
  Bus Creator/1 -> NB/1
  PS-Simulink Converter1/1 -> Bus Creator/2  "pt_x"
  PS-Simulink Converter4/1 -> Bus Creator/5  "vt_y"
  PS-Simulink Converter3/1 -> Bus Creator/3  "pt_y"
  Radians to Degrees/1 -> Bus Creator/1, Scope/1  "ang_wrt_W"
  [TS_theta_RAD] -> Product1/1
  [TS_ax] -> Selector1/1
  Product1/1 -> [TS_SIGNED_theta_RAD]
  Selector1/1 -> Product1/2
  PS-Simulink Converter7/1 -> [TS_theta_RAD]  "ang_wrt_W"
  PS-Simulink Converter8/1 -> [TS_ax]  "TS_ax"
  [TS_SIGNED_theta_RAD] -> Radians to Degrees/1
  connections:
  B/RConn1 -- Transform Sensor/RConn1
  Transform Sensor/LConn1 -- World Frame/RConn1
  Transform Sensor/RConn7 -- PS-Simulink Converter4/LConn1
  PS-Simulink Converter2/LConn1 -- Transform Sensor/RConn6
  PS-Simulink Converter3/LConn1 -- Transform Sensor/RConn5
  PS-Simulink Converter1/LConn1 -- Transform Sensor/RConn4
  PS-Simulink Converter7/LConn1 -- Transform Sensor/RConn2
  PS-Simulink Converter8/LConn1 -- Transform Sensor/RConn3

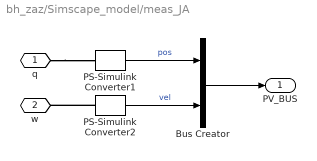
== system bh_zaz/Simscape_model/meas_JA ==
  Bus Creator : BusCreator  Inputs=2
  PS-Simulink Converter1 : nesl_utility/PS-Simulink Converter  PhysicalDomain=network_engine_domain  SubClassName=ps_output  LeftPortType=input  RightPortType=output  PseudoPeriodic=off  Frequencies=[]  Unit=deg  AffineConversion=off
  PS-Simulink Converter2 : nesl_utility/PS-Simulink Converter  PhysicalDomain=network_engine_domain  SubClassName=ps_output  LeftPortType=input  RightPortType=output  PseudoPeriodic=off  Frequencies=[]  Unit=deg/s  AffineConversion=off
  q : PMIOPort  Side=Left
  w : PMIOPort  Port=2  Side=Left
  PV_BUS : Outport  VectorParamsAs1DForOutWhenUnconnected=off
  wires:
  PS-Simulink Converter2/1 -> Bus Creator/2  "vel"
  PS-Simulink Converter1/1 -> Bus Creator/1  "pos"
  Bus Creator/1 -> PV_BUS/1
  connections:
  q/RConn1 -- PS-Simulink Converter1/LConn1
  PS-Simulink Converter2/LConn1 -- w/RConn1

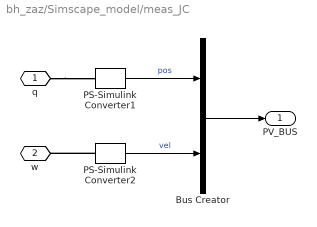
== system bh_zaz/Simscape_model/meas_JC ==
  Bus Creator : BusCreator  Inputs=2
  PS-Simulink Converter1 : nesl_utility/PS-Simulink Converter  PhysicalDomain=network_engine_domain  SubClassName=ps_output  LeftPortType=input  RightPortType=output  PseudoPeriodic=off  Frequencies=[]  Unit=deg  AffineConversion=off
      settings: AttributesFormatString=UNITS=%<Unit>
  PS-Simulink Converter2 : nesl_utility/PS-Simulink Converter  PhysicalDomain=network_engine_domain  SubClassName=ps_output  LeftPortType=input  RightPortType=output  PseudoPeriodic=off  Frequencies=[]  Unit=deg/s  AffineConversion=off
      settings: AttributesFormatString=UNITS=%<Unit>
  q : PMIOPort  Side=Left
  w : PMIOPort  Port=2  Side=Left
  PV_BUS : Outport  VectorParamsAs1DForOutWhenUnconnected=off
  wires:
  PS-Simulink Converter2/1 -> Bus Creator/2  "vel"
  PS-Simulink Converter1/1 -> Bus Creator/1  "pos"
  Bus Creator/1 -> PV_BUS/1
  connections:
  q/RConn1 -- PS-Simulink Converter1/LConn1
  PS-Simulink Converter2/LConn1 -- w/RConn1

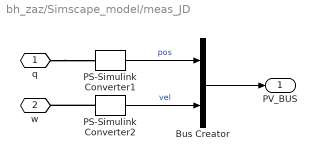
== system bh_zaz/Simscape_model/meas_JD ==
  Bus Creator : BusCreator  Inputs=2
  PS-Simulink Converter1 : nesl_utility/PS-Simulink Converter  PhysicalDomain=network_engine_domain  SubClassName=ps_output  LeftPortType=input  RightPortType=output  PseudoPeriodic=off  Frequencies=[]  Unit=deg  AffineConversion=off
  PS-Simulink Converter2 : nesl_utility/PS-Simulink Converter  PhysicalDomain=network_engine_domain  SubClassName=ps_output  LeftPortType=input  RightPortType=output  PseudoPeriodic=off  Frequencies=[]  Unit=deg/s  AffineConversion=off
  q : PMIOPort  Side=Left
  w : PMIOPort  Port=2  Side=Left
  PV_BUS : Outport  VectorParamsAs1DForOutWhenUnconnected=off
  wires:
  PS-Simulink Converter2/1 -> Bus Creator/2  "vel"
  PS-Simulink Converter1/1 -> Bus Creator/1  "pos"
  Bus Creator/1 -> PV_BUS/1
  connections:
  q/RConn1 -- PS-Simulink Converter1/LConn1
  PS-Simulink Converter2/LConn1 -- w/RConn1
